simulink model "Lab4b"  (R2023a)
settings: Solver=VariableStepAuto  StartTime=0.0  StopTime=0.05  RelTol=1e-3  AbsTol=1e-3
undefined symbols (not defined in the file): Angle, Magnitude
libraries: spsCurrentMeasurementLib x3, spsVoltageMeasurementLib x3, spsLinearTransformerLib x2, spsSeriesRLCBranchLib x2, spsACVoltageSourceLib x1, spspowerguiLib x1
settings Model: Creator=shubh  LastModifiedBy=shubh
settings SolverCC: AutoScaleAbsTol=off  AlgebraicLoopSolver=TrustRegion  MaxZcPerStep=1
settings DebuggingCC: UnconnectedInputMsg=warning  UnconnectedOutputMsg=warning  UnconnectedLineMsg=warning  SymbolicDimsDataTypeCodeGenerationDiagnostic=none
settings ModelReferenceCC: EnableRefExpFcnMdlSchedulingChecks=on
settings SFSimCC: CustomCodeUndefinedFunction=UseInterfaceOnly
settings RTWCC: DLArmComputeVersion=19.05
settings SimscapeCC: SimscapeLogType=all  SimscapeLogSimulationStatistics=on  SimscapeLogDataHistory=10000

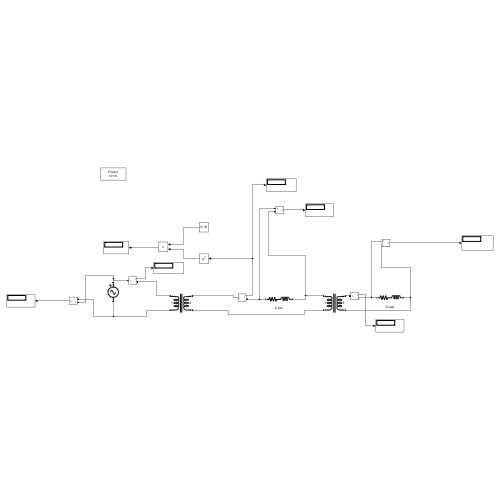
[thumbnail: Simulink's stored preview of the top-level diagram]
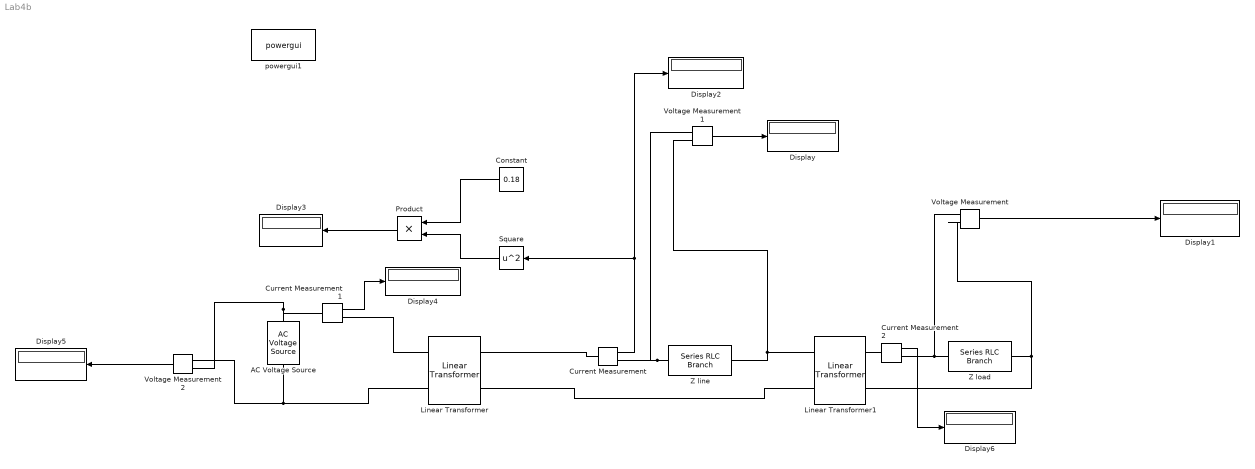
== system Lab4b ==
  AC Voltage Source : spsACVoltageSourceLib/AC Voltage Source  Amplitude=480  Phase=0  Frequency=50  SampleTime=0  Measurements=None  BusType=swing  Pref=10e3  Qref=0  Qmin=-inf  Qmax=+inf
  Constant : Constant  Value=0.18
  Current Measurement : spsCurrentMeasurementLib/Current Measurement  PhasorSimulation=on  OutputType=Magnitude-Angle  PSBequivalent=0
  Current Measurement1 : spsCurrentMeasurementLib/Current Measurement  PhasorSimulation=on  OutputType=Magnitude-Angle  PSBequivalent=0
  Current Measurement2 : spsCurrentMeasurementLib/Current Measurement  PhasorSimulation=on  OutputType=Magnitude-Angle  PSBequivalent=0
  Display{,1..6} (7 alike) : Display
  Linear Transformer : spsLinearTransformerLib/Linear Transformer  UNITS=SI  NominalPower=[ 250e6 50 ]  winding1=[480 0.0001 0.0001]  winding2=[4800 0.0001 0.0001]  ThreeWindings=off  winding3=[3.15e+05 0.7938 0.084225]  RmLm=[1.0804e+06 2866]  Measurements=None  DataType=on
  Linear Transformer1 : spsLinearTransformerLib/Linear Transformer  UNITS=SI  NominalPower=[ 250e6 50 ]  winding1=[4800 0.0001 0.0001]  winding2=[480 0.0001 0.0001]  ThreeWindings=off  winding3=[3.15e+05 0.7938 0.084225]  RmLm=[1.0804e+06 2866]  Measurements=None  DataType=on
  Product : Product
  Square : Math  Operator=square
  Voltage Measurement : spsVoltageMeasurementLib/Voltage Measurement  PhasorSimulation=on  OutputType=Magnitude-Angle  PSBequivalent=0
  Voltage Measurement1 : spsVoltageMeasurementLib/Voltage Measurement  PhasorSimulation=on  OutputType=Magnitude-Angle  PSBequivalent=0
  Voltage Measurement2 : spsVoltageMeasurementLib/Voltage Measurement  PhasorSimulation=on  OutputType=Magnitude-Angle  PSBequivalent=0
  Z line : spsSeriesRLCBranchLib/Series RLC Branch  LConnTagsString=__new0  RConnTagsString=__new0  BranchType=RL  Resistance=0.18  Inductance=0.000764  SetiL0=off  InitialCurrent=0  Capacitance=1e-6  Setx0=off  InitialVoltage=0  Measurements=None
  Z load : spsSeriesRLCBranchLib/Series RLC Branch  LConnTagsString=__new0  RConnTagsString=__new0  BranchType=RL  Resistance=4  Inductance=0.0095  SetiL0=off  InitialCurrent=0  Capacitance=1e-6  Setx0=off  InitialVoltage=0  Measurements=None
  powergui1 : spspowerguiLib/powergui  Priority=1  SimulationMode=Phasor  SampleTime=50e-6  frequency=50  Iterations=50  frequencyindice=50  Pbase=100e6  ErrMax=1e-4  UnitsV=kV  UnitsW=MW  buscounter=0  FunctionMessages=off  echomessages=off  EnableUseOfTLC=off  CurrentSourceSwitches=off  DisableSnubberDevices=off  DisableRonSwitches=off  DisableVfSwitches=off  DisplayEquations=off  AutomaticDiscreteSolvers=off  SolverType=Tustin/Backward Euler (TBE)  Interpol=off  ExternalGateDelay=off  methode=off  Ts=100  x0status=blocks  SPID=on  SwTol=0  HookPort=off  NonlinearTolerance=1e-4  nMaxIteration=100  ContinueOnMaxIteration=off  RestoreLinks=warning  ResistiveCurrentMeasurement=off  Frange=[0:2:500]  Ylog=off  Xlog=on  ShowGrid=off  save=off  variable=ZData  structure=0  ZoomFFT=off  StartTime=0.0  cycles=1  DisplayStyle=1  fundamental=60  FreqAxis=off  MaxFrequency=1000  frequencyindicesteady=1  RmsSteady=1  display=off
  wires:
  Voltage Measurement2/1 -> Display5/1
  Voltage Measurement1/1 -> Display/1
  Constant/1 -> Product/1
  Product/1 -> Display3/1
  Voltage Measurement/1 -> Display1/1
  Square/1 -> Product/2
  Current Measurement/1 -> Display2/1, Square/1
  Current Measurement1/1 -> Display4/1
  Current Measurement2/1 -> Display6/1
  connections:
  Voltage Measurement/LConn2 -- Z load/RConn1 -- Linear Transformer1/RConn2
  Voltage Measurement1/LConn2 -- Z line/RConn1 -- Linear Transformer1/LConn1
  Z line/LConn1 -- Current Measurement/RConn1 -- Voltage Measurement1/LConn1
  AC Voltage Source/RConn1 -- Current Measurement1/LConn1 -- Voltage Measurement2/LConn1
  AC Voltage Source/LConn1 -- Linear Transformer/LConn2 -- Voltage Measurement2/LConn2
  Linear Transformer/RConn1 -- Current Measurement/LConn1
  Linear Transformer/RConn2 -- Linear Transformer1/LConn2
  Current Measurement1/RConn1 -- Linear Transformer/LConn1
  Current Measurement2/LConn1 -- Linear Transformer1/RConn1
  Z load/LConn1 -- Voltage Measurement/LConn1 -- Current Measurement2/RConn1
